simulink model "TUGASuntitled"  (R2014b)
settings: Solver=VariableStepAuto  StartTime=0.0  StopTime=10.0  RelTol=1e-3
values from neighbouring files (symbols this model uses):
  Ab = 4    [12477_Untitled23.m]    (also in 12478_TUGAS2PSDuntitled.slx.m; PSD (2).m)
  L = 1    [12477_Untitled23.m]    (also in 12478_TUGAS2PSDuntitled.slx.m; PSD (2).m)
  Lf = 55    [12477_Untitled23.m]    (also in 12478_TUGAS2PSDuntitled.slx.m; PSD (2).m)
  Lr = 65    [12477_Untitled23.m]    (also in 12478_TUGAS2PSDuntitled.slx.m; PSD (2).m)
  Vo = 20    [12477_Untitled23.m]    (also in 12478_TUGAS2PSDuntitled.slx.m)
libraries: simulink_extras x1
settings Model: Creator=sn10 27.7.17  LastModifiedBy=user
settings DataIOCC: LimitDataPoints=off  SaveFormat=Dataset
settings OptimizationCC: UseDivisionForNetSlopeComputation=off  LifeSpan=auto  SimCompilerOptimization=off
settings DebuggingCC: SolverPrmCheckMsg=none  FcnCallInpInsideContextMsg=error  FrameProcessingCompatibilityMsg=error  SFUnexpectedBacktrackingDiag=error  SFNoUnconditionalDefaultTransitionDiag=error
settings HardwareCC: ProdBitPerPointer=64  ProdLargestAtomicFloat=Float  ProdIntDivRoundTo=Zero  ProdEndianess=LittleEndian  ProdWordSize=64  ProdHWDeviceType=Intel->x86-64 (Windows64)
settings ModelReferenceCC: PropagateSignalLabelsOutOfModel=on
settings RTWCC: RTWCompilerOptimization=off
settings GRTTargetCC: TargetLangStandard=C99 (ISO)  GeneratePreprocessorConditionals=Use local settings

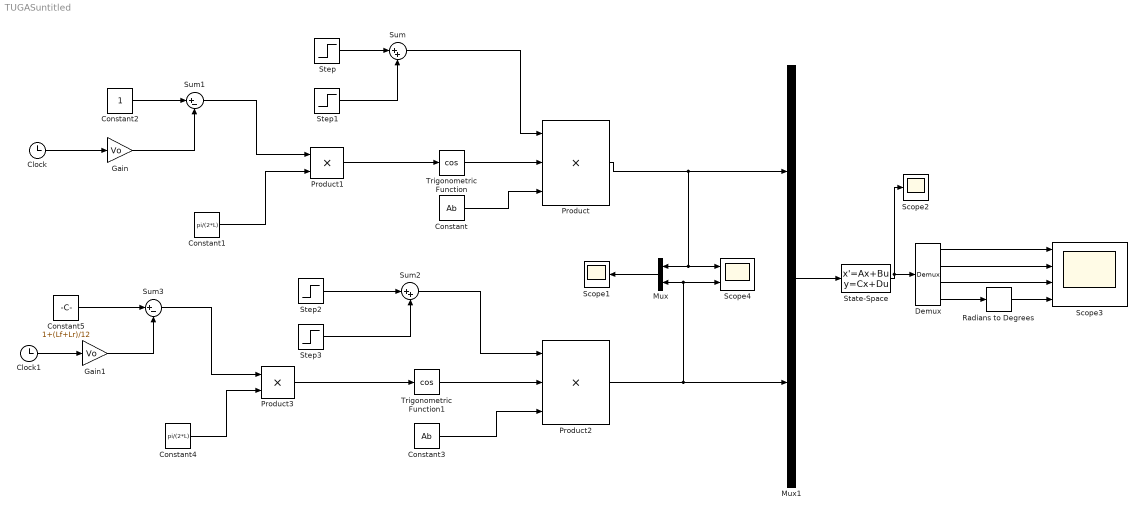
== system TUGASuntitled ==
  Clock : Clock
  Clock1 : Clock
  Constant : Constant  Value=Ab
  Constant1 : Constant  Value=pi/(2*L)
  Constant2 : Constant
  Constant3 : Constant  Value=Ab
  Constant4 : Constant  Value=pi/(2*L)
  Constant5 : Constant  Value=1+(Lf+Lr)/12
  Demux : Demux
  Gain : Gain  Gain=Vo
  Gain1 : Gain  Gain=Vo
  Mux : Mux  Inputs=2
  Mux1 : Mux  Inputs=2
  Product : Product  Inputs=3
  Product1 : Product
  Product2 : Product  Inputs=3
  Product3 : Product
  Radians to Degrees : simulink_extras/Transformations/Radians to Degrees
  Scope1 : Scope
      settings: YMin=-4.99997  YMax=4.99997  SaveName=ScopeData2
  Scope2 : Scope
      settings: YMin=-0.50548  YMax=0.5035  SaveName=ScopeData2
  Scope3 : Scope  NumInputPorts=4
      settings: YMin=-0.00041~-0.48348~-0.50548~-0.54056  YMax=0.00301~0.49775~0.5035~0.53825  SaveName=ScopeData3
  Scope4 : Scope  NumInputPorts=2
      settings: YMin=-4~-4.99403  YMax=4~4.99931
  State-Space : StateSpace  A=[0 1 0 0 0 0 0 0; -1/14 -1/70 1/35 1/168 3/70 1/120 17/14 3/14; 0 0 0 1 0 0 0 0; 24/25 1/5 -244/25 -1/5 0 0 264/5 11; 0 0 0 0 0 1 0 0; 36/25 7/25 0 0 -256/25 -7/25 -468/5 -91/5; 0 0 0 0 0 0 0 1; 51/400 9/400 33/200 11/320 -117/400 -91/1600 -2247/80 -447/80]  B=[0 0; 0 0; 0 0; 44/5 0; 0 0; 0 44/5; 0 0; 0 0]  C=[1 0 0 0 0 0 0 0; 0 0 1 0 0 0 0 0; 0 0 0 0 1 0 0 0; 0 0 0 0 0 0 1 0]  D=[0 0; 0 0; 0 0; 0 0]  X0=0
  Step : Step  Time=0  SampleTime=0
  Step1 : Step  Time=0  Before=1  After=0  SampleTime=0
  Step2 : Step  Time=0  SampleTime=0
  Step3 : Step  Time=0  Before=1  After=0  SampleTime=0
  Sum : Sum  Inputs=|++
  Sum1 : Sum  Inputs=|+-
  Sum2 : Sum  Inputs=|++
  Sum3 : Sum  Inputs=|+-
  Trigonometric Function : Trigonometry  Operator=cos
  Trigonometric Function1 : Trigonometry  Operator=cos
  wires:
  Sum/1 -> Product/1
  Step/1 -> Sum/1
  Step1/1 -> Sum/2
  Trigonometric Function/1 -> Product/2
  Product1/1 -> Trigonometric Function/1
  Constant/1 -> Product/3
  Constant1/1 -> Product1/2
  Sum1/1 -> Product1/1
  Constant2/1 -> Sum1/1
  Gain/1 -> Sum1/2
  Clock/1 -> Gain/1
  Sum2/1 -> Product2/1
  Step2/1 -> Sum2/1
  Step3/1 -> Sum2/2
  Trigonometric Function1/1 -> Product2/2
  Constant3/1 -> Product2/3
  Product3/1 -> Trigonometric Function1/1
  Constant4/1 -> Product3/2
  Sum3/1 -> Product3/1
  Constant5/1 -> Sum3/1
  Gain1/1 -> Sum3/2
  Clock1/1 -> Gain1/1
  Product/1 -> Mux1/1, Scope4/1, Mux/1
  Demux/1 -> Scope3/1
  Demux/2 -> Scope3/2
  Demux/3 -> Scope3/3
  Demux/4 -> Radians to Degrees/1
  State-Space/1 -> Scope2/1, Demux/1
  Product2/1 -> Mux1/2, Scope4/2, Mux/2
  Radians to Degrees/1 -> Scope3/4
  Mux1/1 -> State-Space/1
  Mux/1 -> Scope1/1
